simulink model "MSDRPrimaryLoop_LoadFollow"  (R2021b)
settings: Solver=VariableStepAuto  StartTime=0.0  StopTime=604900  MaxStep=1  MinStep=0.01  RelTol=1e-3
undefined symbols (not defined in the file): a_f, A_free_PHX, a_g, A_h_PHX, beta, beta_t, bubbleGeneratorArea, bubbleGeneratorDh, bubbleGeneratorElevation, bubbleGeneratorLength, bubbleGeneratorVolume, bubbleSaturationLevel, bubbleSeparatorArea, bubbleSeparatorDiameter, bubbleSeparatorDo, bubbleSeparatorLength, bubbleSeparatorSlope, bypassRatio, C0, coreFlowArea, coreFuelVolume, coreLowerPlenumArea, coreLowerPlenumHydraulicDiameter, coreLowerPlenumLength, coreLowerPlenumVolume, coreUpperPlenumArea, coreUpperPlenumHydraulicDiameter, coreUpperPlenumLength, coreUpperPlenumVolume, coreVolume, cpGraphite, dissolusionRatio, dMin, dScale, dsmConst, DXeG, Fiss_factor, fuelChannelHydrualicDiameter, fuelChannelLength, fuelDepositRatio, fuelFraction, fuelGraphiteArea, fuelGraphiteHeatTransferCoefficient, gamma0, gamma1, gamma2, generatorDsm, graphiteKDiff, graphiteUnitCellThickness, initialIodineConcentration, InitialXeMolarConcentration, InjectionRatio, injectionRatio, iodineDecayConstant, IodineDecayConstant, iodineYield, kGraphite, kScale, Lam, lam ... (+60)
libraries: fl_lib x268, nesl_utility x106, SimscapeFluids_lib x20, slpidlib x1
(part 9 of 12)

== system MSDRPrimaryLoop_LoadFollow/Reactor/CoreTH&Inerti/UpperPlenum/UpperPlenum ==
  GasInRef : Inport
  2PModification : Subsystem  ReferencedSubsystem=TwoPhaseModification
      settings: PortSchema="{\"entries\":[{\"content\":{\"sides\":[{\"content\":{\"connectorIds\":[\"LConn1\"]},\"type\":\"ConnectorPlacement.EquallySpacedRectSide\",\"uuid\":\"7546b4b7-b669-49c8-8f27-f696391ea3ad\"},{\"content\":{\"connectorIds\":[\"RConn1\"],\"side\":\"RIGHT\"},\"type\":\"ConnectorPlacement.EquallySpacedRectSide\",\"uuid\":\"0e6176f2-177c-4327-bcfa-9a190fe9083f\"},{\"content\":{\"connectorIds\":[\"LConn2\"],\"side\":\"TOP\"},\"type\":\"ConnectorPlacement.EquallySpacedRectSide\",\"uuid\":\"16faf74c-4635-4009-a5b3-33dd03b625c6\"},{\"content\":{\"connectorIds\":[\"RConn2\",\"In1\"],\"side\":\"BOTTOM\"},\"type\":\"ConnectorPlacement.EquallySpacedRectSide\",\"uuid\":\"2081d73b-bb08-4ad9-b5c8-e48a4e9c4e20\"}]},\"type\":\"ConnectorPlacement.EquallySpacedConnector\",\"uuid\":\"243e4075-206b-4747-a8bc-b8f10d9a577f\"}],\"packageUris\":[\"http://schema.mathworks.com/mf0/Connector/R2020b\"],\"version\":\"1.0\"}"
  PS Abs : fl_lib/Physical Signals/Nonlinear Operators/PS Abs
      settings: SourceProductBaseCode=SS  InternalSimscapePortConfiguration="{\"Bottom\":[],\"Left\":[{\"id\":\"I\",\"label\":\"\",\"type\":\"input\"}],\"Right\":[{\"id\":\"O\",\"label\":\"\",\"type\":\"output\"}],\"Top\":[]}"
  Sudden Area Change (TL)1 : SimscapeFluids_lib/Thermal Liquid/Pipes & Fittings/Sudden Area Change (TL)  loss_spec=fluids.thermal_liquid.enum.area_change_loss_spec.empirical  area_A=coreUpperPlenumArea m^2  area_B=0.005*coreUpperPlenumArea m^2  K_c=1  K_e=1  Re_TLU=[10, 20, 30, 40, 50, 100, 200, 500, 1000, 2000]  loss_contraction_TLU=[5, 2.7, 1.8, 1.46, 1.3, .9, .65, .42, .3, .2]  loss_expansion_TLU=[3.1, 2.3, 1.65, 1.35, 1.15, .9, .75, .65, .9, .65]  length=0.1 m  Re_critical=10
      settings: SourceProductBaseCode=SH  InternalSimscapePortConfiguration="{\"Bottom\":[],\"Left\":[{\"id\":\"A\",\"label\":\"A\",\"type\":\"foundation.thermal_liquid.thermal_liquid\"}],\"Right\":[{\"id\":\"B\",\"label\":\"B\",\"type\":\"foundation.thermal_liquid.thermal_liquid\"}],\"Top\":[]}"
  Sudden Area Change (TL)3 : SimscapeFluids_lib/Thermal Liquid/Pipes & Fittings/Sudden Area Change (TL)  loss_spec=fluids.thermal_liquid.enum.area_change_loss_spec.empirical  area_A=coreUpperPlenumArea m^2  area_B=coreFlowArea m^2  K_c=1  K_e=1  Re_TLU=[10, 20, 30, 40, 50, 100, 200, 500, 1000, 2000]  loss_contraction_TLU=[5, 2.7, 1.8, 1.46, 1.3, .9, .65, .42, .3, .2]  loss_expansion_TLU=[3.1, 2.3, 1.65, 1.35, 1.15, .9, .75, .65, .9, .65]  length=0.1 m  Re_critical=10
      settings: SourceProductBaseCode=SH  InternalSimscapePortConfiguration="{\"Bottom\":[],\"Left\":[{\"id\":\"A\",\"label\":\"A\",\"type\":\"foundation.thermal_liquid.thermal_liquid\"}],\"Right\":[{\"id\":\"B\",\"label\":\"B\",\"type\":\"foundation.thermal_liquid.thermal_liquid\"}],\"Top\":[]}"
  Upper Plenum : SimscapeFluids_lib/Thermal Liquid/Pipes & Fittings/Pipe (TL)  dynamic_compressibility=simscape.enum.onoff.on  inertia=simscape.enum.onoff.off  num_segments=1  pipe_length=coreUpperPlenumVolume/coreUpperPlenumArea m  area=coreUpperPlenumArea m^2  Dh=0.1128 m  wall_spec=fluids.thermal_liquid.pipes_fittings.enum.wall_spec.rigid  Dh_rigid=coreLowerPlenumHydraulicDiameter m  wall_compliance=1.2e-6 m/MPa  wall_time_constant=0.01 s  elevation_spec=foundation.enum.constant_variable.constant  elevation_gain=coreUpperPlenumLength m  g=9.82 m/s^2  pressure_loss_spec=fluids.thermal_liquid.pipes_fittings.enum.PressureLossSpec.Haaland  length_add=1 m  roughness=surfaceRoughness m  Re_friction_TLU=[400, 1000, 1500, 3000, 4000, 6000, 10000, 20000, 40000, 60000, 100000, 100000000]  friction_factor_TLU=[.264, .112, .071, .0417, .0387, .0268, .025, .0232, .0226, .022, .0214, .0214]  shape_factor=64  Re_lam=2000  Re_tur=4000  mdot_nominal=[.1, 1] kg/s  p_diff_nominal=[.001, .01] MPa  mdot_threshold=1e-6 kg/s  heat_transfer_spec=fluids.thermal_liquid.pipes_fittings.enum.HeatTransferSpec.Gnielinski  mdot_nominal_heat=[.1, 1] kg/s  T_in_nominal=[293.15, 293.15] K  T_out_nominal=[300, 300] K  p_in_nominal_heat=[.101325, .101325] MPa  T_wall_nominal=[303.15, 303.15] K  a_coeff=0.023  b_Re_power=0.8  c_Pr_power=0.4  Nu_lam=3.66  Re_Colburn_TLU=[100, 150, 1000]  Colburn_factor_TLU=[.019, .013, .002]  Re_Nu_TLU=[100, 150, 1000]  Pr_Nu_TLU=[1, 10]  Nu_TLU=[3.72, 4.21; 3.75, 4.44; 4.21, 7.15]  T0_vec=T0 K  p0_vec=P0 Pa  mdot0=0.1 kg/s
      settings: SourceProductBaseCode=SH
  Volumetric Flow Rate Sensor (TL) : fl_lib/Thermal Liquid/Sensors/Volumetric Flow Rate Sensor (TL)
      settings: SourceProductBaseCode=SS  InternalSimscapePortConfiguration="{\"Bottom\":[],\"Left\":[{\"id\":\"A\",\"label\":\"A\",\"type\":\"foundation.thermal_liquid.thermal_liquid\"}],\"Right\":[{\"id\":\"B\",\"label\":\"B\",\"type\":\"foundation.thermal_liquid.thermal_liquid\"},{\"id\":\"V\",\"label\":\"V\",\"type\":\"output\"}],\"Top\":[]}"
  Inlet : PMIOPort  Side=Left
  Thermal Connection : PMIOPort  Port=2  Side=Right
  Outlet : PMIOPort  Port=3  Side=Right
  VolumeRate : PMIOPort  Port=4  Side=Right
  wires:
  GasInRef/1 -> 2PModification/1
  connections:
  Volumetric Flow Rate Sensor (TL)/RConn2 -- PS Abs/LConn1
  PS Abs/RConn1 -- VolumeRate/RConn1
  2PModification/RConn1 -- Outlet/RConn1
  2PModification/RConn2 -- Sudden Area Change (TL)1/RConn1 -- 2PModification/LConn1
  2PModification/LConn2 -- Sudden Area Change (TL)3/LConn1 -- Volumetric Flow Rate Sensor (TL)/LConn1
  Volumetric Flow Rate Sensor (TL)/RConn1 -- Upper Plenum/LConn1
  Thermal Connection/RConn1 -- Upper Plenum/LConn2
  Sudden Area Change (TL)3/RConn1 -- Inlet/RConn1
  Upper Plenum/RConn1 -- Sudden Area Change (TL)1/LConn1

== system MSDRPrimaryLoop_LoadFollow/Reactor/CoreTH&Inerti/UpperPlenum/XenonCalc ==
  XeIn : Inport  OutDataTypeStr=double  Unit=kg/s
  PLoss : Inport  Port=2
  GasRef : Inport  Port=3
  Absolute Reference (TL) : fl_lib/Thermal Liquid/Elements/Absolute Reference (TL)
      settings: SourceProductBaseCode=SS
  Demux : Demux  Outputs=2
  Gas : Subsystem
      settings: PortSchema="{\"entries\":[{\"content\":{\"sides\":[{\"content\":{\"connectorIds\":[\"In1\"]},\"type\":\"ConnectorPlacement.EquallySpacedRectSide\",\"uuid\":\"9457d014-8c8c-4ede-953a-dad1b8fcff2e\"},{\"content\":{\"connectorIds\":[\"Out1\"],\"side\":\"RIGHT\"},\"type\":\"ConnectorPlacement.EquallySpacedRectSide\",\"uuid\":\"6b13e550-1648-4662-a58b-f6f49b8dfc45\"},{\"content\":{\"connectorIds\":[\"Out2\",\"In2\"],\"side\":\"TOP\"},\"type\":\"ConnectorPlacement.EquallySpacedRectSide\",\"uuid\":\"73a4211d-b4c2-4f72-9c26-6ee46c1777bd\"},{\"content\":{\"connectorIds\":[\"In3\",\"In4\"],\"side\":\"BOTTOM\"},\"type\":\"ConnectorPlacement.EquallySpacedRectSide\",\"uuid\":\"ca62b0cd-46c8-418f-9a8b-9558726bf444\"}]},\"type\":\"ConnectorPlacement.EquallySpacedConnector\",\"uuid\":\"020f2da1-56fe-4a8a-8a2d-2f75d9123e14\"}],\"packageUris\":[\"http://schema.mathworks.com/mf0/Connector/R2020b\"],\"version\":\"1.0\"}"
  InterphaseTranfser : Subsystem
      settings: PortSchema="{\"entries\":[{\"content\":{\"sides\":[{\"content\":{\"connectorIds\":[\"In1\",\"In2\",\"In3\"]},\"type\":\"ConnectorPlacement.EquallySpacedRectSide\",\"uuid\":\"d6303689-138e-451a-a3c3-60d601b4795c\"},{\"content\":{\"connectorIds\":[\"In5\",\"Out1\"],\"side\":\"RIGHT\"},\"type\":\"ConnectorPlacement.EquallySpacedRectSide\",\"uuid\":\"e99266db-1ad9-4248-a3a9-dc80edd4cbf2\"},{\"content\":{\"connectorIds\":[\"LConn1\"],\"side\":\"TOP\"},\"type\":\"ConnectorPlacement.EquallySpacedRectSide\",\"uuid\":\"07679a3e-e535-452f-8d16-cac9376cf8bb\"},{\"content\":{\"connectorIds\":[\"In4\"],\"side\":\"BOTTOM\"},\"type\":\"ConnectorPlacement.EquallySpacedRectSide\",\"uuid\":\"cd334689-6a33-4cbf-8721-40055306f60f\"}]},\"type\":\"ConnectorPlacement.EquallySpacedConnector\",\"uuid\":\"2a8870ca-366d-4312-85a0-e0a2095078d0\"}],\"packageUris\":[\"http://schema.mathworks.com/mf0/Connector/R2020b\"],\"version\":\"1.0\"}"
  Mux : Mux  Inputs=2
  PS Abs : fl_lib/Physical Signals/Nonlinear Operators/PS Abs
      settings: SourceProductBaseCode=SS  InternalSimscapePortConfiguration="{\"Bottom\":[],\"Left\":[{\"id\":\"I\",\"label\":\"\",\"type\":\"input\"}],\"Right\":[{\"id\":\"O\",\"label\":\"\",\"type\":\"output\"}],\"Top\":[]}"
  PS-Simulink Converter : nesl_utility/PS-Simulink Converter  PhysicalDomain=network_engine_domain  SubClassName=ps_output  LeftPortType=input  RightPortType=output  PseudoPeriodic=off  Frequencies=[]  Unit=inherit  AffineConversion=off
      settings: SourceProductBaseCode=PW,SS
  PS-Simulink Converter1 : nesl_utility/PS-Simulink Converter  PhysicalDomain=network_engine_domain  SubClassName=ps_output  LeftPortType=input  RightPortType=output  PseudoPeriodic=off  Frequencies=[]  Unit=inherit  AffineConversion=off
      settings: SourceProductBaseCode=PW,SS
  Pressure & Temperature Sensor (TL) : fl_lib/Thermal Liquid/Sensors/Pressure & Temperature Sensor (TL)
      settings: SourceProductBaseCode=SS  InternalSimscapePortConfiguration="{\"Bottom\":[],\"Left\":[{\"id\":\"A\",\"label\":\"A\",\"type\":\"foundation.thermal_liquid.thermal_liquid\"}],\"Right\":[{\"id\":\"B\",\"label\":\"B\",\"type\":\"foundation.thermal_liquid.thermal_liquid\"},{\"id\":\"P\",\"label\":\"P\",\"type\":\"output\"},{\"id\":\"T\",\"label\":\"T\",\"type\":\"output\"}],\"Top\":[]}"
  Salt : Subsystem
      settings: PortSchema="{\"entries\":[{\"content\":{\"sides\":[{\"content\":{\"connectorIds\":[\"In1\",\"In2\",\"In3\"]},\"type\":\"ConnectorPlacement.EquallySpacedRectSide\",\"uuid\":\"9457d014-8c8c-4ede-953a-dad1b8fcff2e\"},{\"content\":{\"connectorIds\":[\"Out1\"],\"side\":\"RIGHT\"},\"type\":\"ConnectorPlacement.EquallySpacedRectSide\",\"uuid\":\"6b13e550-1648-4662-a58b-f6f49b8dfc45\"},{\"content\":{\"connectorIds\":[\"In4\",\"In5\"],\"side\":\"TOP\"},\"type\":\"ConnectorPlacement.EquallySpacedRectSide\",\"uuid\":\"73a4211d-b4c2-4f72-9c26-6ee46c1777bd\"},{\"content\":{\"connectorIds\":[\"Out2\",\"In6\"],\"side\":\"BOTTOM\"},\"type\":\"ConnectorPlacement.EquallySpacedRectSide\",\"uuid\":\"ca62b0cd-46c8-418f-9a8b-9558726bf444\"}]},\"type\":\"ConnectorPlacement.EquallySpacedConnector\",\"uuid\":\"020f2da1-56fe-4a8a-8a2d-2f75d9123e14\"}],\"packageUris\":[\"http://schema.mathworks.com/mf0/Connector/R2020b\"],\"version\":\"1.0\"}"
  Volumetric Flow Rate Sensor (TL) : fl_lib/Thermal Liquid/Sensors/Volumetric Flow Rate Sensor (TL)
      settings: SourceProductBaseCode=SS  InternalSimscapePortConfiguration="{\"Bottom\":[],\"Left\":[{\"id\":\"A\",\"label\":\"A\",\"type\":\"foundation.thermal_liquid.thermal_liquid\"}],\"Right\":[{\"id\":\"B\",\"label\":\"B\",\"type\":\"foundation.thermal_liquid.thermal_liquid\"},{\"id\":\"V\",\"label\":\"V\",\"type\":\"output\"}],\"Top\":[]}"
  Inlet : PMIOPort  Side=Left
  Outlet : PMIOPort  Port=2  Side=Right
  XeOut : Outport
  wires:
  XeIn/1 -> Demux/1
  PS-Simulink Converter/1 -> InterphaseTranfser/5(VolumeRate), Gas/4(VolumeRate), Salt/5(VolumeRate)
  GasRef/1 -> Gas/3(GasRef), InterphaseTranfser/2(GasRef), Salt/4(GasRef)
  Demux/1 -> Salt/1(XeLIn)
  [IodineSNDensity] -> Salt/2(IodineSNumberDensity)
  Demux/2 -> Gas/1(XeGIn)
  Salt/1(XeLOut) -> Mux/1
  Gas/1(XeGOut) -> Mux/2
  Mux/1 -> XeOut/1
  Salt/2(GxSalt) -> InterphaseTranfser/1(GxSalt)
  Gas/2(GxGas) -> InterphaseTranfser/3(GxGas)
  InterphaseTranfser/1(TranfserRate) -> Salt/6(Interphase), Gas/2(Interphase)
  PS-Simulink Converter1/1 -> Salt/3(T_f_ave)
  PLoss/1 -> InterphaseTranfser/4(PLoss)
  connections:
  Outlet/RConn1 -- Volumetric Flow Rate Sensor (TL)/RConn1 -- InterphaseTranfser/LConn1
  Volumetric Flow Rate Sensor (TL)/LConn1 -- Pressure & Temperature Sensor (TL)/LConn1 -- Inlet/RConn1
  Volumetric Flow Rate Sensor (TL)/RConn2 -- PS Abs/LConn1
  PS Abs/RConn1 -- PS-Simulink Converter/LConn1
  Pressure & Temperature Sensor (TL)/RConn1 -- Absolute Reference (TL)/LConn1
  Pressure & Temperature Sensor (TL)/RConn3 -- PS-Simulink Converter1/LConn1

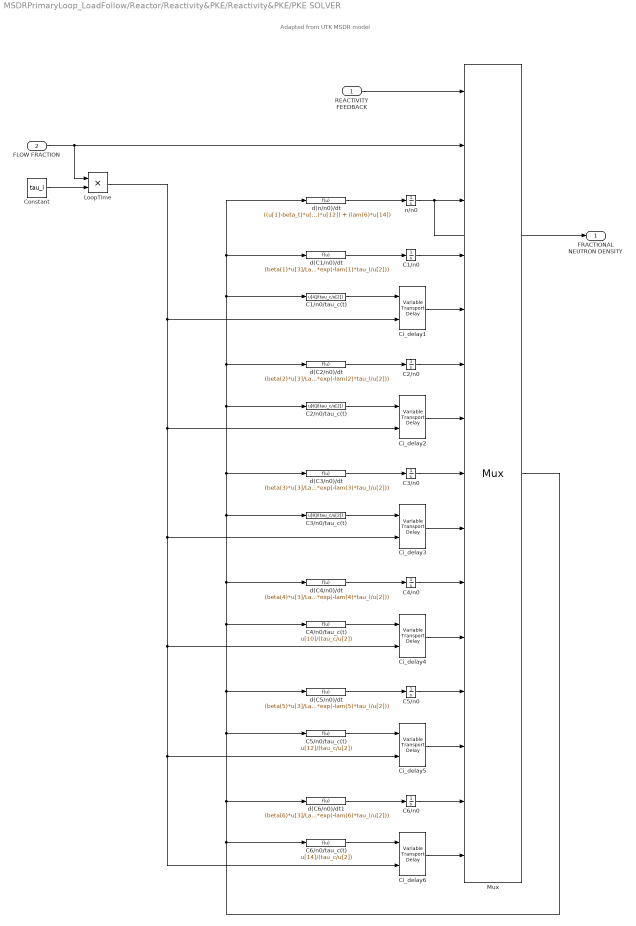
== system MSDRPrimaryLoop_LoadFollow/Reactor/Reactivity&PKE/Reactivity&PKE/PKE SOLVER ==
  note: Adapted from UTK MSDR model
  REACTIVITY FEEDBACK : Inport
  FLOW FRACTION : Inport  Port=2
  C1/n0 : Integrator  InitialCondition=C0(1)
  C1/n0/tau_c(t) : Fcn  Expr=u[4]/(tau_c/u[2])
  C2/n0 : Integrator  InitialCondition=C0(2)
  C2/n0/tau_c(t) : Fcn  Expr=u[6]/(tau_c/u[2])
  C3/n0 : Integrator  InitialCondition=C0(3)
  C3/n0/tau_c(t) : Fcn  Expr=u[8]/(tau_c/u[2])
  C4/n0 : Integrator  InitialCondition=C0(4)
  C4/n0/tau_c(t) : Fcn  Expr=u[10]/(tau_c/u[2])
  C5/n0 : Integrator  InitialCondition=C0(5)
  C5/n0/tau_c(t) : Fcn  Expr=u[12]/(tau_c/u[2])
  C6/n0 : Integrator  InitialCondition=C0(6)
  C6/n0/tau_c(t) : Fcn  Expr=u[14]/(tau_c/u[2])
  Ci_delay1 : VariableTransportDelay  MaximumDelay=1000000  InitialOutput=C0(1)/tau_c
  Ci_delay2 : VariableTransportDelay  MaximumDelay=1000000  InitialOutput=C0(2)/tau_c
  Ci_delay3 : VariableTransportDelay  MaximumDelay=1000000  InitialOutput=C0(3)/tau_c
  Ci_delay4 : VariableTransportDelay  MaximumDelay=1000000  InitialOutput=C0(4)/tau_c
  Ci_delay5 : VariableTransportDelay  MaximumDelay=1000000  InitialOutput=C0(5)/tau_c
  Ci_delay6 : VariableTransportDelay  MaximumDelay=1000000  InitialOutput=C0(6)/tau_c
  Constant : Constant  Value=tau_l
  LoopTime : Product
  Mux : Mux  Inputs=15
      settings: DisplayOption=signals
  d(C1/n0)/dt : Fcn  Expr=(beta(1)*u[3]/Lam) - (lam(1)*u[4]) - (u[4]/(tau_c/u[2])) + (u[5]*exp(-lam(1)*tau_l/u[2]))
  d(C2/n0)/dt : Fcn  Expr=(beta(2)*u[3]/Lam) - (lam(2)*u[6]) - (u[6]/(tau_c/u[2])) + (u[7]*exp(-lam(2)*tau_l/u[2]))
  d(C3/n0)/dt : Fcn  Expr=(beta(3)*u[3]/Lam) - (lam(3)*u[8]) - (u[8]/(tau_c/u[2])) + (u[9]*exp(-lam(3)*tau_l/u[2]))
  d(C4/n0)/dt : Fcn  Expr=(beta(4)*u[3]/Lam) - (lam(4)*u[10]) - (u[10]/(tau_c/u[2])) + (u[11]*exp(-lam(4)*tau_l/u[2]))
  d(C5/n0)/dt : Fcn  Expr=(beta(5)*u[3]/Lam) - (lam(5)*u[12]) - (u[12]/(tau_c/u[2])) + (u[13]*exp(-lam(5)*tau_l/u[2]))
  d(C6/n0)/dt1 : Fcn  Expr=(beta(6)*u[3]/Lam) - (lam(6)*u[14]) - (u[14]/(tau_c/u[2])) + (u[14]*exp(-lam(6)*tau_l/u[2]))
  d(n/n0)/dt : Fcn  Expr=((u[1]-beta_t)*u[3]/Lam) + (lam(1)*u[4]) + (lam(2)*u[6]) + (lam(3)*u[8]) + (lam(4)*u[10]) + (lam(5)*u[12]) + (lam(6)*u[14])
  n/n0 : Integrator  InitialCondition=1
  FRACTIONAL NEUTRON DENSITY : Outport  VectorParamsAs1DForOutWhenUnconnected=off
  wires:
  C1/n0/tau_c(t)/1 -> Ci_delay1/1
  d(n/n0)/dt/1 -> n/n0/1
  d(C1/n0)/dt/1 -> C1/n0/1
  REACTIVITY FEEDBACK/1 -> Mux/1
  n/n0/1 -> FRACTIONAL NEUTRON DENSITY/1, Mux/3
  C1/n0/1 -> Mux/4
  Ci_delay1/1 -> Mux/5
  LoopTime/1 -> Ci_delay6/2, Ci_delay5/2, Ci_delay4/2, Ci_delay3/2, Ci_delay2/2, Ci_delay1/2
  C2/n0/tau_c(t)/1 -> Ci_delay2/1
  d(C2/n0)/dt/1 -> C2/n0/1
  Ci_delay2/1 -> Mux/7
  C2/n0/1 -> Mux/6
  C3/n0/1 -> Mux/8
  d(C3/n0)/dt/1 -> C3/n0/1
  Ci_delay3/1 -> Mux/9
  C3/n0/tau_c(t)/1 -> Ci_delay3/1
  C4/n0/1 -> Mux/10
  C4/n0/tau_c(t)/1 -> Ci_delay4/1
  d(C4/n0)/dt/1 -> C4/n0/1
  Ci_delay4/1 -> Mux/11
  C5/n0/tau_c(t)/1 -> Ci_delay5/1
  d(C5/n0)/dt/1 -> C5/n0/1
  C5/n0/1 -> Mux/12
  Ci_delay5/1 -> Mux/13
  C6/n0/1 -> Mux/14
  d(C6/n0)/dt1/1 -> C6/n0/1
  C6/n0/tau_c(t)/1 -> Ci_delay6/1
  Ci_delay6/1 -> Mux/15
  Mux/1 -> d(n/n0)/dt/1, d(C1/n0)/dt/1, C1/n0/tau_c(t)/1, d(C2/n0)/dt/1, C2/n0/tau_c(t)/1, d(C3/n0)/dt/1, C3/n0/tau_c(t)/1, d(C4/n0)/dt/1, C4/n0/tau_c(t)/1, d(C5/n0)/dt/1, C5/n0/tau_c(t)/1, d(C6/n0)/dt1/1, C6/n0/tau_c(t)/1
  Constant/1 -> LoopTime/2
  FLOW FRACTION/1 -> LoopTime/1, Mux/2

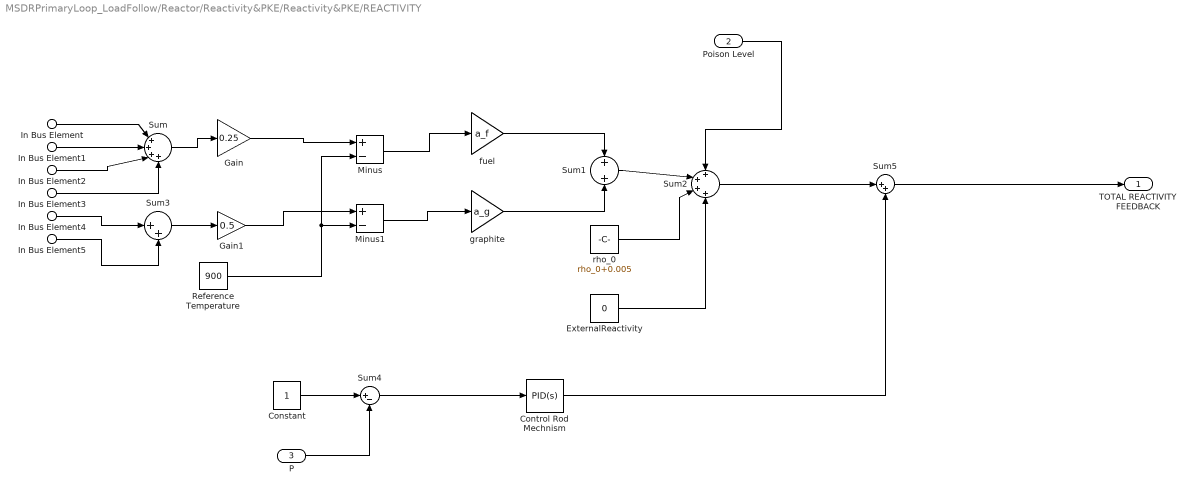
== system MSDRPrimaryLoop_LoadFollow/Reactor/Reactivity&PKE/Reactivity&PKE/REACTIVITY ==
  In Bus Element : Inport  PortName=CORE TEMPERATURE  Element=FuelNode1
  In Bus Element1 : Inport  PortName=CORE TEMPERATURE  Element=FuelNode2
  In Bus Element2 : Inport  PortName=CORE TEMPERATURE  Element=FuelNode3
  In Bus Element3 : Inport  PortName=CORE TEMPERATURE  Element=FuelNode4
  In Bus Element4 : Inport  PortName=CORE TEMPERATURE  Element=GraphiteNode12
  In Bus Element5 : Inport  PortName=CORE TEMPERATURE  Element=GraphiteNode34
  Poison Level : Inport  Port=2
  P : Inport  Port=3
  Constant : Constant
  Control Rod Mechnism : slpidlib/PID Controller  Controller=PID  Form=Parallel  TimeDomain=Continuous-time  UseExternalTs=off  SampleTime=-1  IntegratorMethod=Forward Euler  FilterMethod=Forward Euler  ControllerParametersSource=internal  P=3e-3  I=3e-5  D=3e-3  UseFilter=on  N=100  TunerSelectOption=Transfer Function Based (PID Tuner App)  InitialConditionSource=internal  InitialConditionForIntegrator=0  InitialConditionForFilter=0  DifferentiatorICPrevScaledInput=0  ExternalReset=none  TrackingMode=off  Kt=1  LimitOutput=off  SatLimitsSource=internal  UpperSaturationLimit=inf  LowerSaturationLimit=-inf  LinearizeAsGain=on  AntiWindupMode=none  Kb=1  POutMin=[]  POutMax=[]  IOutMin=[]  IOutMax=[]  DOutMin=[]  DOutMax=[]  NOutMin=[]  NOutMax=[]  SumOutMin=[]  SumOutMax=[]  SaturationOutMin=[]  SaturationOutMax=[]  PParamMin=[]  PParamMax=[]  IParamMin=[]  IParamMax=[]  DParamMin=[]  DParamMax=[]  NParamMin=[]  NParamMax=[]  KbParamMin=[]  KbParamMax=[]  KtParamMin=[]  KtParamMax=[]  KbOutMin=[]  KbOutMax=[]  KtOutMin=[]  KtOutMax=[]  IntegratorOutMin=[]  IntegratorOutMax=[]  FilterOutMin=[]  FilterOutMax=[]  SumI1OutMin=[]  SumI1OutMax=[]  SumI2OutMin=[]  SumI2OutMax=[]  SumI3OutMin=[]  SumI3OutMax=[]  SumI4OutMin=[]  SumI4OutMax=[]  SumDOutMin=[]  SumDOutMax=[]  DifferentiatorOutMin=[]  DifferentiatorOutMax=[]  FilterDiffOutCoefMin=[]  FilterDiffOutCoefMax=[]  ReciprocalOutMin=[]  ReciprocalOutMax=[]  SumDenOutMin=[]  SumDenOutMax=[]  SumNumOutMin=[]  SumNumOutMax=[]  DivideOutMin=[]  DivideOutMax=[]  UdiffTsProdOutMin=[]  UdiffTsProdOutMax=[]  NTsProdOutMin=[]  NTsProdOutMax=[]  UintegralTsProdOutMin=[]  UintegralTsProdOutMax=[]  UngainTsProdOutMin=[]  UngainTsProdOutMax=[]  IntegratorContinuousStateAttributes=''  IntegratorStateMustResolveToSignalObject=off  IntegratorRTWStateStorageClass=Auto  FilterContinuousStateAttributes=''  FilterStateMustResolveToSignalObject=off  FilterRTWStateStorageClass=Auto  ParallelPVariant=InternalParameters  IdealPVariant=Disabled  IVariant=InternalParameters  DVariant=InternalParameters  IntegratorVariant=Continuous  SatVariant=Disabled  AWVariant=Passthrough  PCopyVariant=Disabled  TRVariant=Disabled  FdbkBlocksVariant=Forward  IdealPFdbkVariant=Disabled  SatFdbkVariant=Disabled  DerivativeFilterVariant=ContFilter  NVariant=InternalParameters  NCopyVariant=Disabled  FilterICVariant=InternalICsFilter  IntegratorICVariant=InternalICs  ExternalResetVariant=Disabled  TRSumVariant=Passthrough  SumFdbkVariant=Disabled  SumVariant=Sum_PID  TsampFilterVariant=InternalTs  TsampNgainVariant=Passthrough  TsampIntegralVariant=Passthrough  ExternalSaturationOutDataTypeStr=Inherit: Same as second input
  ExternalReactivity : Constant  Value=0
  Gain : Gain  Gain=0.25
  Gain1 : Gain  Gain=0.5
  Minus : Sum  Inputs=+-
  Minus1 : Sum  Inputs=+-
  Reference Temperature : Constant  Value=900
  Sum : Sum  Inputs=|++++
  Sum1 : Sum
  Sum2 : Sum  Inputs=++++
  Sum3 : Sum  Inputs=|++
  Sum4 : Sum  Inputs=|+-
  Sum5 : Sum  Inputs=|++
  fuel : Gain  Gain=a_f
  graphite : Gain  Gain=a_g
  rho_0 : Constant  Value=rho_0+0.005
  TOTAL REACTIVITY FEEDBACK : Outport  VectorParamsAs1DForOutWhenUnconnected=off
  wires:
  graphite/1 -> Sum1/2
  fuel/1 -> Sum1/1
  Sum1/1 -> Sum2/2
  Poison Level/1 -> Sum2/1
  rho_0/1 -> Sum2/3
  ExternalReactivity/1 -> Sum2/4
  Minus/1 -> fuel/1
  Minus1/1 -> graphite/1
  Reference Temperature/1 -> Minus1/2, Minus/2
  In Bus Element3/1 -> Sum/4
  In Bus Element2/1 -> Sum/3
  In Bus Element1/1 -> Sum/2
  In Bus Element/1 -> Sum/1
  Sum/1 -> Gain/1
  Gain/1 -> Minus/1
  In Bus Element4/1 -> Sum3/1
  In Bus Element5/1 -> Sum3/2
  Sum3/1 -> Gain1/1
  Gain1/1 -> Minus1/1
  Sum4/1 -> Control Rod Mechnism/1
  Sum2/1 -> Sum5/1
  Control Rod Mechnism/1 -> Sum5/2
  Sum5/1 -> TOTAL REACTIVITY FEEDBACK/1
  P/1 -> Sum4/2
  Constant/1 -> Sum4/1

== system MSDRPrimaryLoop_LoadFollow/Reactor/Reactivity&PKE/Reactivity&PKE/Xe and Sm ==
  "XeCore, [cm^2]" : Inport
  NeutronFraction : Inport  Port=2
  Add1 : Sum
  Divide : Product  Inputs=*/
  Nu*TotalFissionCrossSectionInCore : Constant  Value=-nu_pke_235*TotalFissionCrossSection
  Samarium : Subsystem
  Poison Level : Outport  VectorParamsAs1DForOutWhenUnconnected=off
  wires:
  Divide/1 -> Poison Level/1
  Nu*TotalFissionCrossSectionInCore/1 -> Divide/2
  NeutronFraction/1 -> Samarium/1(NeutronFraction)
  Samarium/1("SmInCore, [cm2]") -> Add1/1
  "XeCore, [cm^2]"/1 -> Add1/2
  Add1/1 -> Divide/1

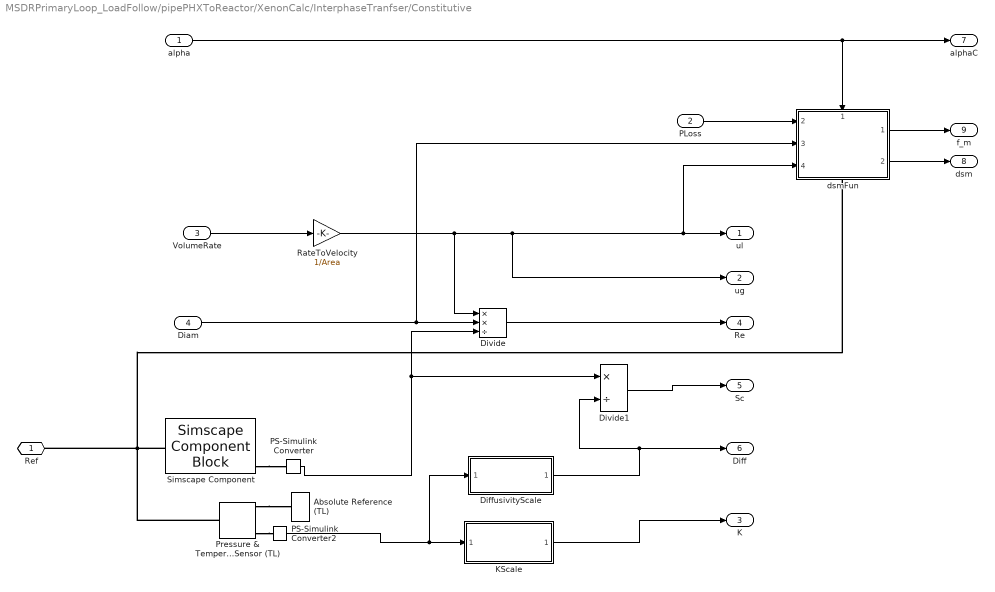
== system MSDRPrimaryLoop_LoadFollow/pipePHXToReactor/XenonCalc/InterphaseTranfser/Constitutive ==
  alpha : Inport
  PLoss : Inport  Port=2
  VolumeRate : Inport  Port=3
  Diam : Inport  Port=4
  Absolute Reference (TL) : fl_lib/Thermal Liquid/Elements/Absolute Reference (TL)
      settings: SourceProductBaseCode=SS
  DiffusivityScale : Subsystem  ReferencedSubsystem=DiffusivityScale
  Divide : Product  Inputs=**/
  Divide1 : Product  Inputs=*/
  KScale : Subsystem  ReferencedSubsystem=KScale
  PS-Simulink Converter : nesl_utility/PS-Simulink Converter  PhysicalDomain=network_engine_domain  SubClassName=ps_output  LeftPortType=input  RightPortType=output  PseudoPeriodic=off  Frequencies=[]  Unit=inherit  AffineConversion=off
      settings: SourceProductBaseCode=PW,SS
  PS-Simulink Converter2 : nesl_utility/PS-Simulink Converter  PhysicalDomain=network_engine_domain  SubClassName=ps_output  LeftPortType=input  RightPortType=output  PseudoPeriodic=off  Frequencies=[]  Unit=inherit  AffineConversion=off
      settings: SourceProductBaseCode=PW,SS
  Pressure & Temperature Sensor (TL) : fl_lib/Thermal Liquid/Sensors/Pressure & Temperature Sensor (TL)
      settings: SourceProductBaseCode=SS  InternalSimscapePortConfiguration="{\"Bottom\":[],\"Left\":[{\"id\":\"A\",\"label\":\"A\",\"type\":\"foundation.thermal_liquid.thermal_liquid\"}],\"Right\":[{\"id\":\"B\",\"label\":\"B\",\"type\":\"foundation.thermal_liquid.thermal_liquid\"},{\"id\":\"P\",\"label\":\"P\",\"type\":\"output\"},{\"id\":\"T\",\"label\":\"T\",\"type\":\"output\"}],\"Top\":[]}"
  RateToVelocity : Gain  Gain=1/Area
  Simscape Component : SimscapeComponentBlock  SourceFile=TL_FullSensor  ComponentPath=TL_FullSensor  ComponentVariants="[\"TL_FullSensor\"]"  ComponentVariantNames="[\"TL_FullSensor\"]"  ClassName=TL_FullSensor  SchemaVersion=1
      settings: CopyFcn=simscape.engine.sli.internal.componentblockcallback(gcbh,'COPY')  PreCopyFcn=simscape.engine.sli.internal.componentblockcallback(gcbh,'PRECOPY')  PreDeleteFcn=simscape.engine.sli.internal.componentblockcallback(gcbh,'PREDELETE')  InternalSimscapePortConfiguration="{\"Bottom\":[],\"Left\":[{\"id\":\"A\",\"label\":\"A\",\"type\":\"foundation.thermal_liquid.thermal_liquid\"}],\"Right\":[{\"id\":\"U\",\"label\":\"u\",\"type\":\"output\"},{\"id\":\"RHO\",\"label\":\"rho\",\"type\":\"output\"},{\"id\":\"CP\",\"label\":\"cp\",\"type\":\"output\"},{\"id\":\"NU\",\"label\":\"nu\",\"type\":\"output\"}],\"Top\":[]}"
      mask Type: Thermodynamic Properties Sensor (TL)
  dsmFun : Subsystem  ReferencedSubsystem=dsmFun
      settings: PortSchema="{\"entries\":[{\"content\":{\"sides\":[{\"content\":{\"connectorIds\":[\"In2\",\"In3\",\"In4\"]},\"type\":\"ConnectorPlacement.EquallySpacedRectSide\",\"uuid\":\"cd878d6d-d881-48a3-8bcf-2f6377bc2619\"},{\"content\":{\"connectorIds\":[\"Out1\",\"Out2\"],\"side\":\"RIGHT\"},\"type\":\"ConnectorPlacement.EquallySpacedRectSide\",\"uuid\":\"84ec48cd-6af4-419c-aaeb-7134212c3ae2\"},{\"content\":{\"connectorIds\":[\"In1\"],\"side\":\"TOP\"},\"type\":\"ConnectorPlacement.EquallySpacedRectSide\",\"uuid\":\"d836bcb8-c56c-40d6-b9ba-0790b759147b\"},{\"content\":{\"connectorIds\":[\"RConn1\"],\"side\":\"BOTTOM\"},\"type\":\"ConnectorPlacement.EquallySpacedRectSide\",\"uuid\":\"16763d39-53e3-4dc4-9c8a-2531c5df2d8d\"}]},\"type\":\"ConnectorPlacement.EquallySpacedConnector\",\"uuid\":\"ad3a93fd-9624-45a3-bd6b-21e42fcd018d\"}],\"packageUris\":[\"http://schema.mathworks.com/mf0/Connector/R2020b\"],\"version\":\"1.0\"}"
  Ref : PMIOPort  Side=Left
  ul : Outport
  ug : Outport  Port=2
  K : Outport  Port=3
  Re : Outport  Port=4
  Sc : Outport  Port=5
  Diff : Outport  Port=6
  alphaC : Outport  Port=7
  dsm : Outport  Port=8
  f_m : Outport  Port=9
  wires:
  alpha/1 -> alphaC/1, dsmFun/1
  VolumeRate/1 -> RateToVelocity/1
  RateToVelocity/1 -> ug/1, dsmFun/4, ul/1, Divide/1
  Diam/1 -> Divide/2, dsmFun/3
  PS-Simulink Converter/1 -> Divide/3, Divide1/1
  PS-Simulink Converter2/1 -> DiffusivityScale/1, KScale/1
  DiffusivityScale/1 -> Divide1/2, Diff/1
  Divide1/1 -> Sc/1
  KScale/1 -> K/1
  dsmFun/2 -> dsm/1
  Divide/1 -> Re/1
  dsmFun/1 -> f_m/1
  PLoss/1 -> dsmFun/2
  connections:
  Pressure & Temperature Sensor (TL)/LConn1 -- dsmFun/RConn1 -- Simscape Component/LConn1 -- Ref/RConn1
  Simscape Component/RConn4 -- PS-Simulink Converter/LConn1
  Pressure & Temperature Sensor (TL)/RConn3 -- PS-Simulink Converter2/LConn1
  Pressure & Temperature Sensor (TL)/RConn1 -- Absolute Reference (TL)/LConn1

== system MSDRPrimaryLoop_LoadFollow/pipePHXToReactor/XenonCalc/Salt/InPipeGeneration ==
  IodineSNumberDensity : Inport
  T_f_ave : Inport  Port=2
  DecayXenonGenerationRate : Product
  Molar/s : Product  Inputs=*/
  Na : Constant  Value=6.022e23
  T2Rho : Fcn  Expr=3960 - 0.6724*u
  gain : Gain  Gain=iodineDecayConstant*Volume
  kg/s : Gain  Gain=0.135
  "XenonGenerationRate, [kg/s]" : Outport
  wires:
  IodineSNumberDensity/1 -> gain/1
  gain/1 -> DecayXenonGenerationRate/1
  T_f_ave/1 -> T2Rho/1
  DecayXenonGenerationRate/1 -> Molar/s/1
  Na/1 -> Molar/s/2
  Molar/s/1 -> kg/s/1
  kg/s/1 -> "XenonGenerationRate, [kg/s]"/1
  T2Rho/1 -> DecayXenonGenerationRate/2

== system MSDRPrimaryLoop_LoadFollow/pipePHXToReactor/XenonCalc/Salt/Subsystem1 ==
  Gas : Inport
  Add1 : Sum  Inputs=+-
  Constant : Constant
  Subsystem : Subsystem  ReferencedSubsystem=GasToAlpha
  1-alpha : Outport
  wires:
  Gas/1 -> Subsystem/1
  Constant/1 -> Add1/1
  Subsystem/1 -> Add1/2
  Add1/1 -> 1-alpha/1

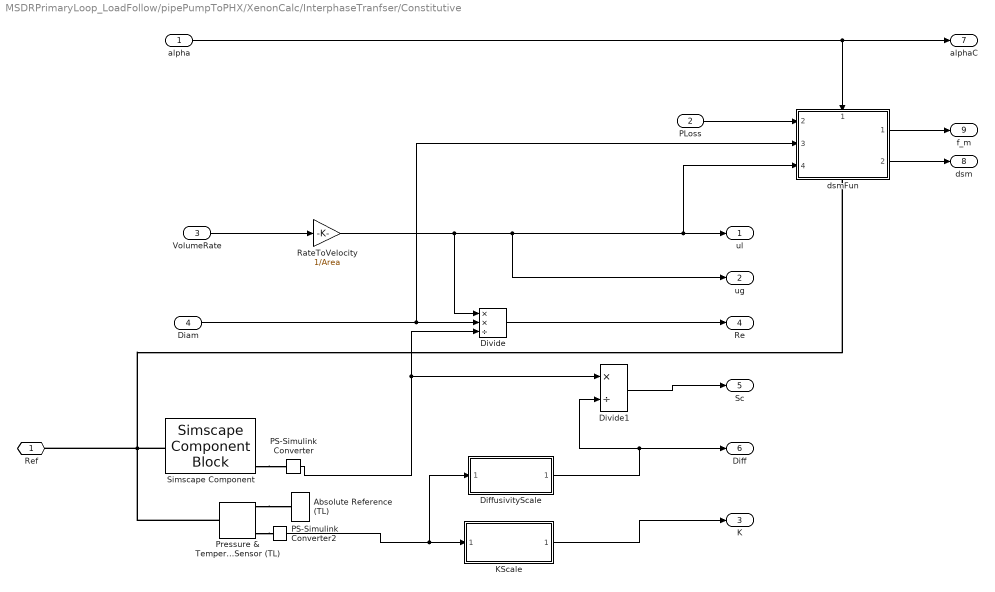
== system MSDRPrimaryLoop_LoadFollow/pipePumpToPHX/XenonCalc/InterphaseTranfser/Constitutive ==
  alpha : Inport
  PLoss : Inport  Port=2
  VolumeRate : Inport  Port=3
  Diam : Inport  Port=4
  Absolute Reference (TL) : fl_lib/Thermal Liquid/Elements/Absolute Reference (TL)
      settings: SourceProductBaseCode=SS
  DiffusivityScale : Subsystem  ReferencedSubsystem=DiffusivityScale
  Divide : Product  Inputs=**/
  Divide1 : Product  Inputs=*/
  KScale : Subsystem  ReferencedSubsystem=KScale
  PS-Simulink Converter : nesl_utility/PS-Simulink Converter  PhysicalDomain=network_engine_domain  SubClassName=ps_output  LeftPortType=input  RightPortType=output  PseudoPeriodic=off  Frequencies=[]  Unit=inherit  AffineConversion=off
      settings: SourceProductBaseCode=PW,SS
  PS-Simulink Converter2 : nesl_utility/PS-Simulink Converter  PhysicalDomain=network_engine_domain  SubClassName=ps_output  LeftPortType=input  RightPortType=output  PseudoPeriodic=off  Frequencies=[]  Unit=inherit  AffineConversion=off
      settings: SourceProductBaseCode=PW,SS
  Pressure & Temperature Sensor (TL) : fl_lib/Thermal Liquid/Sensors/Pressure & Temperature Sensor (TL)
      settings: SourceProductBaseCode=SS  InternalSimscapePortConfiguration="{\"Bottom\":[],\"Left\":[{\"id\":\"A\",\"label\":\"A\",\"type\":\"foundation.thermal_liquid.thermal_liquid\"}],\"Right\":[{\"id\":\"B\",\"label\":\"B\",\"type\":\"foundation.thermal_liquid.thermal_liquid\"},{\"id\":\"P\",\"label\":\"P\",\"type\":\"output\"},{\"id\":\"T\",\"label\":\"T\",\"type\":\"output\"}],\"Top\":[]}"
  RateToVelocity : Gain  Gain=1/Area
  Simscape Component : SimscapeComponentBlock  SourceFile=TL_FullSensor  ComponentPath=TL_FullSensor  ComponentVariants="[\"TL_FullSensor\"]"  ComponentVariantNames="[\"TL_FullSensor\"]"  ClassName=TL_FullSensor  SchemaVersion=1
      settings: CopyFcn=simscape.engine.sli.internal.componentblockcallback(gcbh,'COPY')  PreCopyFcn=simscape.engine.sli.internal.componentblockcallback(gcbh,'PRECOPY')  PreDeleteFcn=simscape.engine.sli.internal.componentblockcallback(gcbh,'PREDELETE')  InternalSimscapePortConfiguration="{\"Bottom\":[],\"Left\":[{\"id\":\"A\",\"label\":\"A\",\"type\":\"foundation.thermal_liquid.thermal_liquid\"}],\"Right\":[{\"id\":\"U\",\"label\":\"u\",\"type\":\"output\"},{\"id\":\"RHO\",\"label\":\"rho\",\"type\":\"output\"},{\"id\":\"CP\",\"label\":\"cp\",\"type\":\"output\"},{\"id\":\"NU\",\"label\":\"nu\",\"type\":\"output\"}],\"Top\":[]}"
      mask Type: Thermodynamic Properties Sensor (TL)
  dsmFun : Subsystem  ReferencedSubsystem=dsmFun
      settings: PortSchema="{\"entries\":[{\"content\":{\"sides\":[{\"content\":{\"connectorIds\":[\"In2\",\"In3\",\"In4\"]},\"type\":\"ConnectorPlacement.EquallySpacedRectSide\",\"uuid\":\"cd878d6d-d881-48a3-8bcf-2f6377bc2619\"},{\"content\":{\"connectorIds\":[\"Out1\",\"Out2\"],\"side\":\"RIGHT\"},\"type\":\"ConnectorPlacement.EquallySpacedRectSide\",\"uuid\":\"84ec48cd-6af4-419c-aaeb-7134212c3ae2\"},{\"content\":{\"connectorIds\":[\"In1\"],\"side\":\"TOP\"},\"type\":\"ConnectorPlacement.EquallySpacedRectSide\",\"uuid\":\"d836bcb8-c56c-40d6-b9ba-0790b759147b\"},{\"content\":{\"connectorIds\":[\"RConn1\"],\"side\":\"BOTTOM\"},\"type\":\"ConnectorPlacement.EquallySpacedRectSide\",\"uuid\":\"16763d39-53e3-4dc4-9c8a-2531c5df2d8d\"}]},\"type\":\"ConnectorPlacement.EquallySpacedConnector\",\"uuid\":\"ad3a93fd-9624-45a3-bd6b-21e42fcd018d\"}],\"packageUris\":[\"http://schema.mathworks.com/mf0/Connector/R2020b\"],\"version\":\"1.0\"}"
  Ref : PMIOPort  Side=Left
  ul : Outport
  ug : Outport  Port=2
  K : Outport  Port=3
  Re : Outport  Port=4
  Sc : Outport  Port=5
  Diff : Outport  Port=6
  alphaC : Outport  Port=7
  dsm : Outport  Port=8
  f_m : Outport  Port=9
  wires:
  alpha/1 -> alphaC/1, dsmFun/1
  VolumeRate/1 -> RateToVelocity/1
  RateToVelocity/1 -> ug/1, dsmFun/4, ul/1, Divide/1
  Diam/1 -> Divide/2, dsmFun/3
  PS-Simulink Converter/1 -> Divide/3, Divide1/1
  PS-Simulink Converter2/1 -> DiffusivityScale/1, KScale/1
  DiffusivityScale/1 -> Divide1/2, Diff/1
  Divide1/1 -> Sc/1
  KScale/1 -> K/1
  dsmFun/2 -> dsm/1
  Divide/1 -> Re/1
  dsmFun/1 -> f_m/1
  PLoss/1 -> dsmFun/2
  connections:
  Pressure & Temperature Sensor (TL)/LConn1 -- dsmFun/RConn1 -- Simscape Component/LConn1 -- Ref/RConn1
  Simscape Component/RConn4 -- PS-Simulink Converter/LConn1
  Pressure & Temperature Sensor (TL)/RConn3 -- PS-Simulink Converter2/LConn1
  Pressure & Temperature Sensor (TL)/RConn1 -- Absolute Reference (TL)/LConn1

== system MSDRPrimaryLoop_LoadFollow/pipePumpToPHX/XenonCalc/Salt/InPipeGeneration ==
  IodineSNumberDensity : Inport
  T_f_ave : Inport  Port=2
  DecayXenonGenerationRate : Product
  Molar/s : Product  Inputs=*/
  Na : Constant  Value=6.022e23
  T2Rho : Fcn  Expr=3960 - 0.6724*u
  gain : Gain  Gain=iodineDecayConstant*Volume
  kg/s : Gain  Gain=0.135
  "XenonGenerationRate, [kg/s]" : Outport
  wires:
  IodineSNumberDensity/1 -> gain/1
  T_f_ave/1 -> T2Rho/1
  gain/1 -> DecayXenonGenerationRate/1
  T2Rho/1 -> DecayXenonGenerationRate/2
  DecayXenonGenerationRate/1 -> Molar/s/1
  Na/1 -> Molar/s/2
  Molar/s/1 -> kg/s/1
  kg/s/1 -> "XenonGenerationRate, [kg/s]"/1

== system MSDRPrimaryLoop_LoadFollow/pipePumpToPHX/XenonCalc/Salt/Subsystem1 ==
  Gas : Inport
  Add1 : Sum  Inputs=+-
  Constant : Constant
  Subsystem : Subsystem  ReferencedSubsystem=GasToAlpha
  1-alpha : Outport
  wires:
  Gas/1 -> Subsystem/1
  Constant/1 -> Add1/1
  Subsystem/1 -> Add1/2
  Add1/1 -> 1-alpha/1

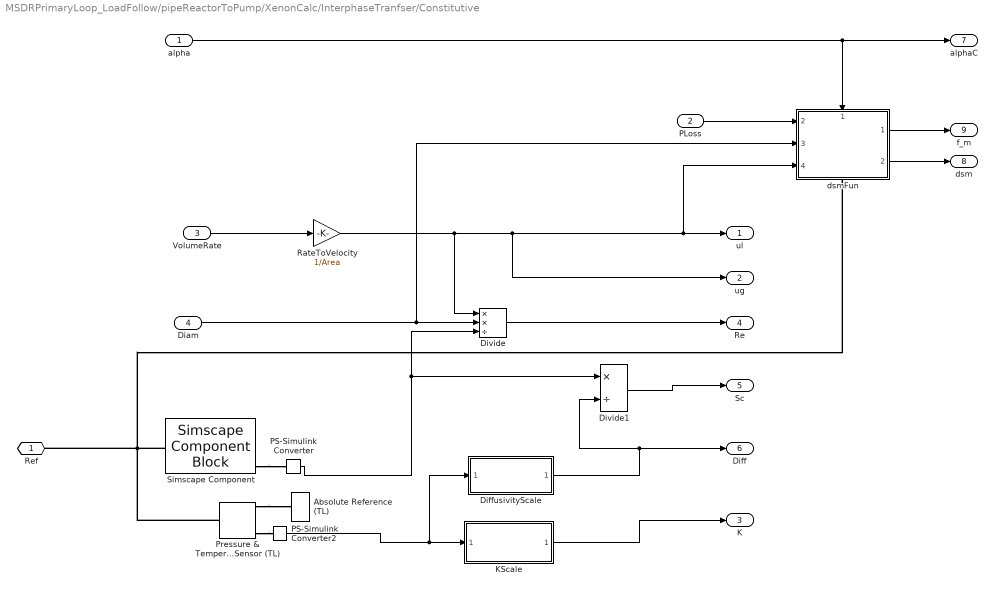
== system MSDRPrimaryLoop_LoadFollow/pipeReactorToPump/XenonCalc/InterphaseTranfser/Constitutive ==
  alpha : Inport
  PLoss : Inport  Port=2
  VolumeRate : Inport  Port=3
  Diam : Inport  Port=4
  Absolute Reference (TL) : fl_lib/Thermal Liquid/Elements/Absolute Reference (TL)
      settings: SourceProductBaseCode=SS
  DiffusivityScale : Subsystem  ReferencedSubsystem=DiffusivityScale
  Divide : Product  Inputs=**/
  Divide1 : Product  Inputs=*/
  KScale : Subsystem  ReferencedSubsystem=KScale
  PS-Simulink Converter : nesl_utility/PS-Simulink Converter  PhysicalDomain=network_engine_domain  SubClassName=ps_output  LeftPortType=input  RightPortType=output  PseudoPeriodic=off  Frequencies=[]  Unit=inherit  AffineConversion=off
      settings: SourceProductBaseCode=PW,SS
  PS-Simulink Converter2 : nesl_utility/PS-Simulink Converter  PhysicalDomain=network_engine_domain  SubClassName=ps_output  LeftPortType=input  RightPortType=output  PseudoPeriodic=off  Frequencies=[]  Unit=inherit  AffineConversion=off
      settings: SourceProductBaseCode=PW,SS
  Pressure & Temperature Sensor (TL) : fl_lib/Thermal Liquid/Sensors/Pressure & Temperature Sensor (TL)
      settings: SourceProductBaseCode=SS  InternalSimscapePortConfiguration="{\"Bottom\":[],\"Left\":[{\"id\":\"A\",\"label\":\"A\",\"type\":\"foundation.thermal_liquid.thermal_liquid\"}],\"Right\":[{\"id\":\"B\",\"label\":\"B\",\"type\":\"foundation.thermal_liquid.thermal_liquid\"},{\"id\":\"P\",\"label\":\"P\",\"type\":\"output\"},{\"id\":\"T\",\"label\":\"T\",\"type\":\"output\"}],\"Top\":[]}"
  RateToVelocity : Gain  Gain=1/Area
  Simscape Component : SimscapeComponentBlock  SourceFile=TL_FullSensor  ComponentPath=TL_FullSensor  ComponentVariants="[\"TL_FullSensor\"]"  ComponentVariantNames="[\"TL_FullSensor\"]"  ClassName=TL_FullSensor  SchemaVersion=1
      settings: CopyFcn=simscape.engine.sli.internal.componentblockcallback(gcbh,'COPY')  PreCopyFcn=simscape.engine.sli.internal.componentblockcallback(gcbh,'PRECOPY')  PreDeleteFcn=simscape.engine.sli.internal.componentblockcallback(gcbh,'PREDELETE')  InternalSimscapePortConfiguration="{\"Bottom\":[],\"Left\":[{\"id\":\"A\",\"label\":\"A\",\"type\":\"foundation.thermal_liquid.thermal_liquid\"}],\"Right\":[{\"id\":\"U\",\"label\":\"u\",\"type\":\"output\"},{\"id\":\"RHO\",\"label\":\"rho\",\"type\":\"output\"},{\"id\":\"CP\",\"label\":\"cp\",\"type\":\"output\"},{\"id\":\"NU\",\"label\":\"nu\",\"type\":\"output\"}],\"Top\":[]}"
      mask Type: Thermodynamic Properties Sensor (TL)
  dsmFun : Subsystem  ReferencedSubsystem=dsmFun
      settings: PortSchema="{\"entries\":[{\"content\":{\"sides\":[{\"content\":{\"connectorIds\":[\"In2\",\"In3\",\"In4\"]},\"type\":\"ConnectorPlacement.EquallySpacedRectSide\",\"uuid\":\"cd878d6d-d881-48a3-8bcf-2f6377bc2619\"},{\"content\":{\"connectorIds\":[\"Out1\",\"Out2\"],\"side\":\"RIGHT\"},\"type\":\"ConnectorPlacement.EquallySpacedRectSide\",\"uuid\":\"84ec48cd-6af4-419c-aaeb-7134212c3ae2\"},{\"content\":{\"connectorIds\":[\"In1\"],\"side\":\"TOP\"},\"type\":\"ConnectorPlacement.EquallySpacedRectSide\",\"uuid\":\"d836bcb8-c56c-40d6-b9ba-0790b759147b\"},{\"content\":{\"connectorIds\":[\"RConn1\"],\"side\":\"BOTTOM\"},\"type\":\"ConnectorPlacement.EquallySpacedRectSide\",\"uuid\":\"16763d39-53e3-4dc4-9c8a-2531c5df2d8d\"}]},\"type\":\"ConnectorPlacement.EquallySpacedConnector\",\"uuid\":\"ad3a93fd-9624-45a3-bd6b-21e42fcd018d\"}],\"packageUris\":[\"http://schema.mathworks.com/mf0/Connector/R2020b\"],\"version\":\"1.0\"}"
  Ref : PMIOPort  Side=Left
  ul : Outport
  ug : Outport  Port=2
  K : Outport  Port=3
  Re : Outport  Port=4
  Sc : Outport  Port=5
  Diff : Outport  Port=6
  alphaC : Outport  Port=7
  dsm : Outport  Port=8
  f_m : Outport  Port=9
  wires:
  alpha/1 -> alphaC/1, dsmFun/1
  VolumeRate/1 -> RateToVelocity/1
  RateToVelocity/1 -> ug/1, dsmFun/4, ul/1, Divide/1
  Diam/1 -> Divide/2, dsmFun/3
  PS-Simulink Converter/1 -> Divide/3, Divide1/1
  PS-Simulink Converter2/1 -> DiffusivityScale/1, KScale/1
  DiffusivityScale/1 -> Divide1/2, Diff/1
  Divide1/1 -> Sc/1
  KScale/1 -> K/1
  dsmFun/2 -> dsm/1
  Divide/1 -> Re/1
  dsmFun/1 -> f_m/1
  PLoss/1 -> dsmFun/2
  connections:
  Pressure & Temperature Sensor (TL)/LConn1 -- dsmFun/RConn1 -- Simscape Component/LConn1 -- Ref/RConn1
  Simscape Component/RConn4 -- PS-Simulink Converter/LConn1
  Pressure & Temperature Sensor (TL)/RConn3 -- PS-Simulink Converter2/LConn1
  Pressure & Temperature Sensor (TL)/RConn1 -- Absolute Reference (TL)/LConn1

== system MSDRPrimaryLoop_LoadFollow/pipeReactorToPump/XenonCalc/Salt/InPipeGeneration ==
  IodineSNumberDensity : Inport
  T_f_ave : Inport  Port=2
  DecayXenonGenerationRate : Product
  Molar/s : Product  Inputs=*/
  Na : Constant  Value=6.022e23
  T2Rho : Fcn  Expr=3960 - 0.6724*u
  gain : Gain  Gain=iodineDecayConstant*Volume
  kg/s : Gain  Gain=0.135
  "XenonGenerationRate, [kg/s]" : Outport
  wires:
  IodineSNumberDensity/1 -> gain/1
  T_f_ave/1 -> T2Rho/1
  gain/1 -> DecayXenonGenerationRate/1
  T2Rho/1 -> DecayXenonGenerationRate/2
  DecayXenonGenerationRate/1 -> Molar/s/1
  Na/1 -> Molar/s/2
  Molar/s/1 -> kg/s/1
  kg/s/1 -> "XenonGenerationRate, [kg/s]"/1

== system MSDRPrimaryLoop_LoadFollow/pipeReactorToPump/XenonCalc/Salt/Subsystem1 ==
  Gas : Inport
  Add1 : Sum  Inputs=+-
  Constant : Constant
  Subsystem : Subsystem  ReferencedSubsystem=GasToAlpha
  1-alpha : Outport
  wires:
  Gas/1 -> Subsystem/1
  Constant/1 -> Add1/1
  Subsystem/1 -> Add1/2
  Add1/1 -> 1-alpha/1

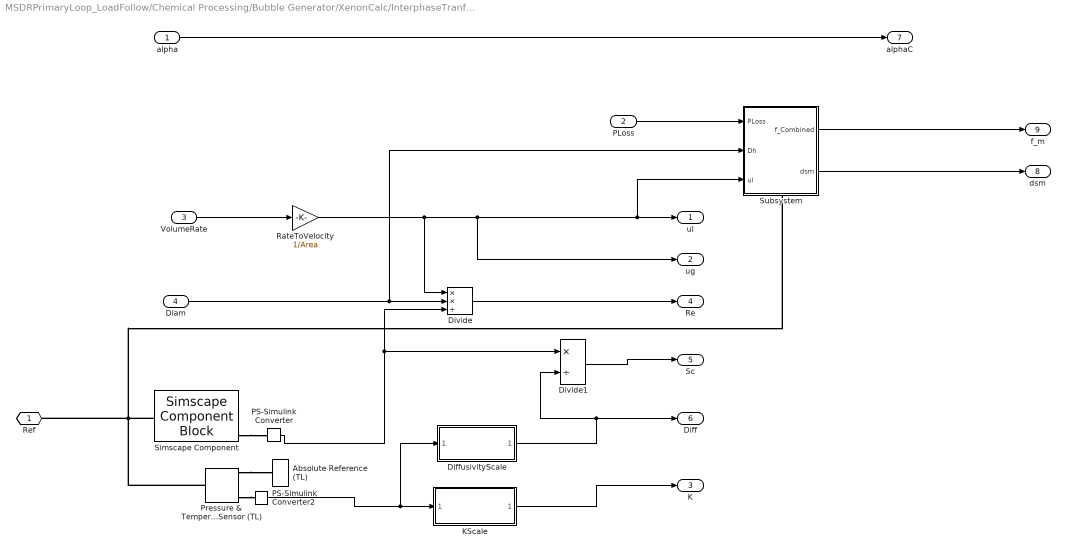
== system MSDRPrimaryLoop_LoadFollow/Chemical Processing/Bubble Generator/XenonCalc/InterphaseTranfser/Constitutive ==
  alpha : Inport
  PLoss : Inport  Port=2
  VolumeRate : Inport  Port=3
  Diam : Inport  Port=4
  Absolute Reference (TL) : fl_lib/Thermal Liquid/Elements/Absolute Reference (TL)
      settings: SourceProductBaseCode=SS
  DiffusivityScale : Subsystem  ReferencedSubsystem=DiffusivityScale
  Divide : Product  Inputs=**/
  Divide1 : Product  Inputs=*/
  KScale : Subsystem  ReferencedSubsystem=KScale
  PS-Simulink Converter : nesl_utility/PS-Simulink Converter  PhysicalDomain=network_engine_domain  SubClassName=ps_output  LeftPortType=input  RightPortType=output  PseudoPeriodic=off  Frequencies=[]  Unit=inherit  AffineConversion=off
      settings: SourceProductBaseCode=PW,SS
  PS-Simulink Converter2 : nesl_utility/PS-Simulink Converter  PhysicalDomain=network_engine_domain  SubClassName=ps_output  LeftPortType=input  RightPortType=output  PseudoPeriodic=off  Frequencies=[]  Unit=inherit  AffineConversion=off
      settings: SourceProductBaseCode=PW,SS
  Pressure & Temperature Sensor (TL) : fl_lib/Thermal Liquid/Sensors/Pressure & Temperature Sensor (TL)
      settings: SourceProductBaseCode=SS  InternalSimscapePortConfiguration="{\"Bottom\":[],\"Left\":[{\"id\":\"A\",\"label\":\"A\",\"type\":\"foundation.thermal_liquid.thermal_liquid\"}],\"Right\":[{\"id\":\"B\",\"label\":\"B\",\"type\":\"foundation.thermal_liquid.thermal_liquid\"},{\"id\":\"P\",\"label\":\"P\",\"type\":\"output\"},{\"id\":\"T\",\"label\":\"T\",\"type\":\"output\"}],\"Top\":[]}"
  RateToVelocity : Gain  Gain=1/Area
  Simscape Component : SimscapeComponentBlock  SourceFile=TL_FullSensor  ComponentPath=TL_FullSensor  ComponentVariants="[\"TL_FullSensor\"]"  ComponentVariantNames="[\"TL_FullSensor\"]"  ClassName=TL_FullSensor  SchemaVersion=1
      settings: CopyFcn=simscape.engine.sli.internal.componentblockcallback(gcbh,'COPY')  PreCopyFcn=simscape.engine.sli.internal.componentblockcallback(gcbh,'PRECOPY')  PreDeleteFcn=simscape.engine.sli.internal.componentblockcallback(gcbh,'PREDELETE')  InternalSimscapePortConfiguration="{\"Bottom\":[],\"Left\":[{\"id\":\"A\",\"label\":\"A\",\"type\":\"foundation.thermal_liquid.thermal_liquid\"}],\"Right\":[{\"id\":\"U\",\"label\":\"u\",\"type\":\"output\"},{\"id\":\"RHO\",\"label\":\"rho\",\"type\":\"output\"},{\"id\":\"CP\",\"label\":\"cp\",\"type\":\"output\"},{\"id\":\"NU\",\"label\":\"nu\",\"type\":\"output\"}],\"Top\":[]}"
      mask Type: Thermodynamic Properties Sensor (TL)
  Subsystem : Subsystem
      settings: PortSchema="{\"entries\":[{\"content\":{\"sides\":[{\"content\":{\"connectorIds\":[\"In1\",\"In2\",\"In3\"]},\"type\":\"ConnectorPlacement.EquallySpacedRectSide\",\"uuid\":\"dd1c86c2-327e-41b5-90e0-a07cc4f7a239\"},{\"content\":{\"connectorIds\":[\"Out1\",\"Out2\"],\"side\":\"RIGHT\"},\"type\":\"ConnectorPlacement.EquallySpacedRectSide\",\"uuid\":\"1daff71e-8b5d-4f35-9ce7-352085350762\"},{\"content\":{\"connectorIds\":[],\"side\":\"TOP\"},\"type\":\"ConnectorPlacement.EquallySpacedRectSide\",\"uuid\":\"6cf7e847-c1ca-4561-96b9-90e4339d236b\"},{\"content\":{\"connectorIds\":[\"RConn1\"],\"side\":\"BOTTOM\"},\"type\":\"ConnectorPlacement.EquallySpacedRectSide\",\"uuid\":\"444ecab7-0e05-438f-8395-0556f9cb1910\"}]},\"type\":\"ConnectorPlacement.EquallySpacedConnector\",\"uuid\":\"a820de5e-57ef-4a78-919f-756fbb4a48db\"}],\"packageUris\":[\"http://schema.mathworks.com/mf0/Connector/R2020b\"],\"version\":\"1.0\"}"
  Ref : PMIOPort  Side=Left
  ul : Outport
  ug : Outport  Port=2
  K : Outport  Port=3
  Re : Outport  Port=4
  Sc : Outport  Port=5
  Diff : Outport  Port=6
  alphaC : Outport  Port=7
  dsm : Outport  Port=8
  f_m : Outport  Port=9
  wires:
  alpha/1 -> alphaC/1
  VolumeRate/1 -> RateToVelocity/1
  RateToVelocity/1 -> ug/1, Subsystem/3(ul), ul/1, Divide/1
  Diam/1 -> Subsystem/2(Dh), Divide/2
  PS-Simulink Converter/1 -> Divide/3, Divide1/1
  PS-Simulink Converter2/1 -> DiffusivityScale/1, KScale/1
  DiffusivityScale/1 -> Divide1/2, Diff/1
  Divide1/1 -> Sc/1
  KScale/1 -> K/1
  Subsystem/2(dsm) -> dsm/1
  Divide/1 -> Re/1
  Subsystem/1(f_Combined) -> f_m/1
  PLoss/1 -> Subsystem/1(PLoss)
  connections:
  Pressure & Temperature Sensor (TL)/LConn1 -- Simscape Component/LConn1 -- Ref/RConn1 -- Subsystem/RConn1
  Simscape Component/RConn4 -- PS-Simulink Converter/LConn1
  Pressure & Temperature Sensor (TL)/RConn3 -- PS-Simulink Converter2/LConn1
  Pressure & Temperature Sensor (TL)/RConn1 -- Absolute Reference (TL)/LConn1

== system MSDRPrimaryLoop_LoadFollow/Chemical Processing/Bubble Generator/XenonCalc/Salt/InPipeGeneration ==
  IodineSNumberDensity : Inport
  T_f_ave : Inport  Port=2
  DecayXenonGenerationRate : Product
  Molar/s : Product  Inputs=*/
  Na : Constant  Value=6.022e23
  T2Rho : Fcn  Expr=3960 - 0.6724*u
  gain : Gain  Gain=iodineDecayConstant*Volume
  kg/s : Gain  Gain=0.135
  "XenonGenerationRate, [kg/s]" : Outport
  wires:
  IodineSNumberDensity/1 -> gain/1
  T_f_ave/1 -> T2Rho/1
  gain/1 -> DecayXenonGenerationRate/1
  T2Rho/1 -> DecayXenonGenerationRate/2
  DecayXenonGenerationRate/1 -> Molar/s/1
  Na/1 -> Molar/s/2
  Molar/s/1 -> kg/s/1
  kg/s/1 -> "XenonGenerationRate, [kg/s]"/1

== system MSDRPrimaryLoop_LoadFollow/Chemical Processing/Bubble Generator/XenonCalc/Salt/Subsystem1 ==
  Gas : Inport
  Add1 : Sum  Inputs=+-
  Constant : Constant
  Subsystem : Subsystem  ReferencedSubsystem=GasToAlpha
  1-alpha : Outport
  wires:
  Gas/1 -> Subsystem/1
  Constant/1 -> Add1/1
  Subsystem/1 -> Add1/2
  Add1/1 -> 1-alpha/1

== system MSDRPrimaryLoop_LoadFollow/Chemical Processing/Bubble Separator/Subsystem/Constitutive/Subsystem ==
  Constant2 : Constant  Value=generatorDsm
  dsm : Outport
  wires:
  Constant2/1 -> dsm/1

== system MSDRPrimaryLoop_LoadFollow/Chemical Processing/ElevationPipe/XenonCalc/InterphaseTranfser1/Constitutive ==
  alpha : Inport
  PLoss : Inport  Port=2
  VolumeRate : Inport  Port=3
  Diam : Inport  Port=4
  Absolute Reference (TL) : fl_lib/Thermal Liquid/Elements/Absolute Reference (TL)
      settings: SourceProductBaseCode=SS
  DiffusivityScale : Subsystem  ReferencedSubsystem=DiffusivityScale
  Divide : Product  Inputs=**/
  Divide1 : Product  Inputs=*/
  KScale : Subsystem  ReferencedSubsystem=KScale
  PS-Simulink Converter : nesl_utility/PS-Simulink Converter  PhysicalDomain=network_engine_domain  SubClassName=ps_output  LeftPortType=input  RightPortType=output  PseudoPeriodic=off  Frequencies=[]  Unit=inherit  AffineConversion=off
      settings: SourceProductBaseCode=PW,SS
  PS-Simulink Converter2 : nesl_utility/PS-Simulink Converter  PhysicalDomain=network_engine_domain  SubClassName=ps_output  LeftPortType=input  RightPortType=output  PseudoPeriodic=off  Frequencies=[]  Unit=inherit  AffineConversion=off
      settings: SourceProductBaseCode=PW,SS
  Pressure & Temperature Sensor (TL) : fl_lib/Thermal Liquid/Sensors/Pressure & Temperature Sensor (TL)
      settings: SourceProductBaseCode=SS  InternalSimscapePortConfiguration="{\"Bottom\":[],\"Left\":[{\"id\":\"A\",\"label\":\"A\",\"type\":\"foundation.thermal_liquid.thermal_liquid\"}],\"Right\":[{\"id\":\"B\",\"label\":\"B\",\"type\":\"foundation.thermal_liquid.thermal_liquid\"},{\"id\":\"P\",\"label\":\"P\",\"type\":\"output\"},{\"id\":\"T\",\"label\":\"T\",\"type\":\"output\"}],\"Top\":[]}"
  RateToVelocity : Gain  Gain=1/Area
  Simscape Component : SimscapeComponentBlock  SourceFile=TL_FullSensor  ComponentPath=TL_FullSensor  ComponentVariants="[\"TL_FullSensor\"]"  ComponentVariantNames="[\"TL_FullSensor\"]"  ClassName=TL_FullSensor  SchemaVersion=1
      settings: CopyFcn=simscape.engine.sli.internal.componentblockcallback(gcbh,'COPY')  PreCopyFcn=simscape.engine.sli.internal.componentblockcallback(gcbh,'PRECOPY')  PreDeleteFcn=simscape.engine.sli.internal.componentblockcallback(gcbh,'PREDELETE')  InternalSimscapePortConfiguration="{\"Bottom\":[],\"Left\":[{\"id\":\"A\",\"label\":\"A\",\"type\":\"foundation.thermal_liquid.thermal_liquid\"}],\"Right\":[{\"id\":\"U\",\"label\":\"u\",\"type\":\"output\"},{\"id\":\"RHO\",\"label\":\"rho\",\"type\":\"output\"},{\"id\":\"CP\",\"label\":\"cp\",\"type\":\"output\"},{\"id\":\"NU\",\"label\":\"nu\",\"type\":\"output\"}],\"Top\":[]}"
      mask Type: Thermodynamic Properties Sensor (TL)
  Subsystem : Subsystem
      settings: PortSchema="{\"entries\":[{\"content\":{\"sides\":[{\"content\":{\"connectorIds\":[\"In1\",\"In2\",\"In3\"]},\"type\":\"ConnectorPlacement.EquallySpacedRectSide\",\"uuid\":\"dd1c86c2-327e-41b5-90e0-a07cc4f7a239\"},{\"content\":{\"connectorIds\":[\"Out1\",\"Out2\"],\"side\":\"RIGHT\"},\"type\":\"ConnectorPlacement.EquallySpacedRectSide\",\"uuid\":\"1daff71e-8b5d-4f35-9ce7-352085350762\"},{\"content\":{\"connectorIds\":[],\"side\":\"TOP\"},\"type\":\"ConnectorPlacement.EquallySpacedRectSide\",\"uuid\":\"6cf7e847-c1ca-4561-96b9-90e4339d236b\"},{\"content\":{\"connectorIds\":[\"RConn1\"],\"side\":\"BOTTOM\"},\"type\":\"ConnectorPlacement.EquallySpacedRectSide\",\"uuid\":\"444ecab7-0e05-438f-8395-0556f9cb1910\"}]},\"type\":\"ConnectorPlacement.EquallySpacedConnector\",\"uuid\":\"a820de5e-57ef-4a78-919f-756fbb4a48db\"}],\"packageUris\":[\"http://schema.mathworks.com/mf0/Connector/R2020b\"],\"version\":\"1.0\"}"
  Ref : PMIOPort  Side=Left
  ul : Outport
  ug : Outport  Port=2
  K : Outport  Port=3
  Re : Outport  Port=4
  Sc : Outport  Port=5
  Diff : Outport  Port=6
  alphaC : Outport  Port=7
  dsm : Outport  Port=8
  f_m : Outport  Port=9
  wires:
  alpha/1 -> alphaC/1
  VolumeRate/1 -> RateToVelocity/1
  RateToVelocity/1 -> ug/1, Subsystem/3(ul), ul/1, Divide/1
  Diam/1 -> Subsystem/2(Dh), Divide/2
  PS-Simulink Converter/1 -> Divide/3, Divide1/1
  PS-Simulink Converter2/1 -> DiffusivityScale/1, KScale/1
  DiffusivityScale/1 -> Divide1/2, Diff/1
  Divide1/1 -> Sc/1
  KScale/1 -> K/1
  Subsystem/2(dsm) -> dsm/1
  Divide/1 -> Re/1
  Subsystem/1(f_Combined) -> f_m/1
  PLoss/1 -> Subsystem/1(PLoss)
  connections:
  Pressure & Temperature Sensor (TL)/LConn1 -- Simscape Component/LConn1 -- Ref/RConn1 -- Subsystem/RConn1
  Simscape Component/RConn4 -- PS-Simulink Converter/LConn1
  Pressure & Temperature Sensor (TL)/RConn3 -- PS-Simulink Converter2/LConn1
  Pressure & Temperature Sensor (TL)/RConn1 -- Absolute Reference (TL)/LConn1

== system MSDRPrimaryLoop_LoadFollow/Chemical Processing/ElevationPipe/XenonCalc/Salt/InPipeGeneration ==
  IodineSNumberDensity : Inport
  T_f_ave : Inport  Port=2
  DecayXenonGenerationRate : Product
  Molar/s : Product  Inputs=*/
  Na : Constant  Value=6.022e23
  T2Rho : Fcn  Expr=3960 - 0.6724*u
  gain : Gain  Gain=iodineDecayConstant*Volume
  kg/s : Gain  Gain=0.135
  "XenonGenerationRate, [kg/s]" : Outport
  wires:
  IodineSNumberDensity/1 -> gain/1
  T_f_ave/1 -> T2Rho/1
  gain/1 -> DecayXenonGenerationRate/1
  T2Rho/1 -> DecayXenonGenerationRate/2
  DecayXenonGenerationRate/1 -> Molar/s/1
  Na/1 -> Molar/s/2
  Molar/s/1 -> kg/s/1
  kg/s/1 -> "XenonGenerationRate, [kg/s]"/1

== system MSDRPrimaryLoop_LoadFollow/Chemical Processing/ElevationPipe/XenonCalc/Salt/Subsystem1 ==
  Gas : Inport
  Add1 : Sum  Inputs=+-
  Constant : Constant
  Subsystem : Subsystem  ReferencedSubsystem=GasToAlpha
  1-alpha : Outport
  wires:
  Gas/1 -> Subsystem/1
  Constant/1 -> Add1/1
  Subsystem/1 -> Add1/2
  Add1/1 -> 1-alpha/1
